simulink model "TVModel"  (R2022a)
settings: Solver=FixedStepDiscrete  StartTime=0.0  StopTime=10.0  FixedStep=0.02  MaxStep=0.01  RelTol=1e-3
undefined symbols (not defined in the file or in its folder): MB, TV, TV_OLD
libraries: simulink x22, simulink_extras x14, slpidlib x8, fuzblock x5, controlLib x4, dspstat3 x4, eeGeneralControl x3, cstblocks x3, eeSlidingModeController x1, sharedTrackingLibrary x1
(part 7 of 8)

== system TVModel/Subsystem/Subsystem1/Torque Distribution/MPC/States Constraints/Tire Bound Dynamics/Slip Angle Calculation/Slip Angle RL ==
  In Bus Element : Inport  PortName=dynamics_data  Element=vy
  In Bus Element1 : Inport  PortName=dynamics_data  Element=vx
  In Bus Element2 : Inport  PortName=dynamics_data  Element=yaw_rate
  In Bus Element3 : Inport  PortName=dynamics_data  Element=yaw_rate
  Atan : Trigonometry  Operator=atan2
  Gain : Gain  Gain=TV.CAR.b
  Gain1 : Gain  Gain=TV.CAR.tr/2
  Subtract : Sum  Inputs=+-
  Subtract1 : Sum  Inputs=+-
  alpha_rl : Outport
  wires:
  In Bus Element2/1 -> Gain/1
  In Bus Element/1 -> Subtract1/1
  In Bus Element3/1 -> Gain1/1
  In Bus Element1/1 -> Subtract/1
  Subtract1/1 -> Atan/1
  Atan/1 -> alpha_rl/1
  Gain1/1 -> Subtract/2
  Gain/1 -> Subtract1/2
  Subtract/1 -> Atan/2

== system TVModel/Subsystem/Subsystem1/Torque Distribution/MPC/States Constraints/Tire Bound Dynamics/Slip Angle Calculation/Slip Angle RR ==
  In Bus Element : Inport  PortName=dynamics_data  Element=vy
  In Bus Element1 : Inport  PortName=dynamics_data  Element=vx
  In Bus Element2 : Inport  PortName=dynamics_data  Element=yaw_rate
  In Bus Element4 : Inport  PortName=dynamics_data  Element=yaw_rate
  Atan : Trigonometry  Operator=atan2
  Gain : Gain  Gain=TV.CAR.b
  Gain1 : Gain  Gain=TV.CAR.tr/2
  Subtract : Sum
  Subtract1 : Sum  Inputs=+-
  alpha_rr : Outport
  wires:
  In Bus Element4/1 -> Gain/1
  In Bus Element/1 -> Subtract1/1
  In Bus Element2/1 -> Gain1/1
  In Bus Element1/1 -> Subtract/1
  Subtract1/1 -> Atan/1
  Atan/1 -> alpha_rr/1
  Gain1/1 -> Subtract/2
  Gain/1 -> Subtract1/2
  Subtract/1 -> Atan/2

== system TVModel/Subsystem/Subsystem1/Torque Distribution/MPC/USEFUL STUFFFF/Power flag/Efficiency limit/Power to engines ==
  omega_motor : Inport
  Torque : Inport  Port=2
  2-D Lookup Table : Lookup_n-D  BreakpointsForDimension1=TV.LV.efficiency_LUT.Omega  BreakpointsForDimension2=TV.LV.efficiency_LUT.Torque  Table=TV.LV.efficiency_LUT.Eta  InternalRulePriority=Speed  RndMeth=Simplest
      settings: InputPortMap=u0,u1
  Abs : Abs  SaturateOnIntegerOverflow=off
  Saturation : Saturate  UpperLimit=1  LowerLimit=0.3
  Efficiency : Outport
  wires:
  Abs/1 -> 2-D Lookup Table/2
  omega_motor/1 -> 2-D Lookup Table/1  "[rad/s]"
  Saturation/1 -> Efficiency/1  "eta_22"
  2-D Lookup Table/1 -> Saturation/1
  Torque/1 -> Abs/1

== system TVModel/Subsystem/Subsystem1/Torque Distribution/MPC/USEFUL STUFFFF/Subsystem1/Steer Activation/First Activation ==
  In1 : Inport
  AND1 : Logic  IconShape=distinctive  AllPortsSameDT=off  OutDataTypeStr=boolean
  Constant9 : Constant  Value=0
  Less Than3 : RelationalOperator  Operator===  OutDataTypeStr=boolean  RndMeth=Simplest  InputSameDT=off
  Less Than4 : RelationalOperator  Operator=<  OutDataTypeStr=boolean  RndMeth=Simplest  InputSameDT=off
  Unit Delay1 : UnitDelay  SampleTime=-1  HasFrameUpgradeWarning=on
  Out1 : Outport
  wires:
  Constant9/1 -> Less Than3/2, Less Than4/1
  Unit Delay1/1 -> Less Than3/1
  In1/1 -> Less Than4/2, Unit Delay1/1
  Less Than4/1 -> AND1/2
  Less Than3/1 -> AND1/1
  AND1/1 -> Out1/1

== system TVModel/Subsystem/Subsystem1/Torque Distribution/MPC/USEFUL STUFFFF/Subsystem1/Steer Activation/If Action Subsystem ==
  Inport : Inport
  Action Port : ActionPort
  Data Type Conversion : DataTypeConversion  OutDataTypeStr=double  RndMeth=Nearest  SaturateOnIntegerOverflow=off
  Epsilon : Outport
  wires:
  Inport/1 -> Data Type Conversion/1
  Data Type Conversion/1 -> Epsilon/1

== system TVModel/Subsystem/Subsystem1/Torque Distribution/MPC/USEFUL STUFFFF/Subsystem1/Steer Activation/If Action Subsystem1 ==
  Inport : Inport
  Action Port : ActionPort
  Constant : Constant  Value=1*pi/180
  Gain : Gain  Gain=1/(2*pi/180)
  Saturation : Saturate  UpperLimit=1  LowerLimit=0
  Saturation1 : Saturate  UpperLimit=inf  LowerLimit=0
  Subtract : Sum  Inputs=+-
  epsilon : Outport
  wires:
  Saturation1/1 -> Gain/1
  Saturation/1 -> epsilon/1
  Gain/1 -> Saturation/1
  Subtract/1 -> Saturation1/1
  Inport/1 -> Subtract/1
  Constant/1 -> Subtract/2

== system TVModel/Subsystem/Subsystem1/Torque Distribution/MPC/ PRE LUDO/Faul Detection/Vectorino/Vectorino/30//70 ==
  In1 : Inport
  Constant2 : Constant  Value=TV.LV.TORQUE.T_peak_motor*[0.3;0.3;1;1]
  Product : Product
  Out1 : Outport
  wires:
  In1/1 -> Product/1
  Product/1 -> Out1/1
  Constant2/1 -> Product/2

== system TVModel/Subsystem/Subsystem1/Torque Distribution/MPC/ PRE LUDO/Faul Detection/Vectorino/Vectorino/Vectorino ==
  In Bus Element4 : Inport  PortName=driver_inputs  Element=steering
  In Bus Element1 : Inport  PortName=driver_inputs  Element=throttle
  In Bus Element : Inport  Port=2  PortName=dynamics_data  Element=omega_wheels
  In Bus Element32 : Inport  Port=3  PortName=brake_signal
  If Action Subsystem2 : Subsystem  TreatAsAtomicUnit=on
  Omega wheels : Subsystem
  Saturation : Saturate  UpperLimit=+inf  LowerLimit=0
  Out Bus Element : Outport  PortName=TV
  wires:
  In Bus Element/1 -> Omega wheels/1(vehBUS)
  In Bus Element1/1 -> If Action Subsystem2/3(Thr)
  In Bus Element32/1 -> If Action Subsystem2/4(Brake)
  Saturation/1 -> If Action Subsystem2/2(Omega wheels)
  In Bus Element4/1 -> If Action Subsystem2/1(delta)
  Omega wheels/1(omega wheels) -> Saturation/1
  If Action Subsystem2/1(T vectorino) -> Out Bus Element/1

== system TVModel/Subsystem/Subsystem1/Torque Distribution/MPC/Faults Detection/Vectorino/Vectorino/Vectorino/If Action Subsystem2 ==
  In Bus Element2 : Inport  PortName=delta
  In Bus Element : Inport  Port=2  PortName=Omega wheels
  In Bus Element1 : Inport  Port=2  PortName=Omega wheels
  In Bus Element5 : Inport  Port=3  PortName=Thr
  In Bus Element3 : Inport  Port=4  PortName=Brake
  In Bus Element4 : Inport  Port=4  PortName=Brake
  If : If  IfExpression=u1 < 0.001
  If Action Subsystem : Subsystem  TreatAsAtomicUnit=on
  If Action Subsystem1 : Subsystem  TreatAsAtomicUnit=on
  Lateral Distribution : Subsystem
  Longitudinal Distribution : Subsystem
  Merge : Merge
  Regen : Subsystem
  T vectorino : Outport
  wires:
  Merge/1 -> T vectorino/1
  If/2 -> If Action Subsystem1/Action
  If/1 -> If Action Subsystem/Action
  In Bus Element2/1 -> Lateral Distribution/2(delta)
  Lateral Distribution/1(TV) -> If Action Subsystem/1(T TV)
  Longitudinal Distribution/1(Front Axle Torque) -> Lateral Distribution/1(Front Axle Torque)
  In Bus Element5/1 -> Longitudinal Distribution/1(Throttle)
  Longitudinal Distribution/2(" Rear Axle Torque") -> Lateral Distribution/3(Rear Axle Torque)
  Regen/1(TV) -> If Action Subsystem1/1(T vectorino)
  If Action Subsystem/1(T_out) -> Merge/1
  If Action Subsystem1/1(T regen) -> Merge/2
  In Bus Element/1 -> Regen/1(Omega wheels)
  In Bus Element1/1 -> Lateral Distribution/4(omega wheels)
  In Bus Element3/1 -> Regen/2(Brake)
  In Bus Element4/1 -> If/1

== system TVModel/Subsystem/Subsystem1/Torque Distribution/MPC/Faults Detection/Vectorino/Vectorino/Vectorino/Omega wheels ==
  In Bus Element : Inport  PortName=vehBUS  Element=Dir.Powertrain.FR.Motor.Velocity
  In Bus Element1 : Inport  PortName=vehBUS  Element=Dir.Powertrain.FL.Motor.Velocity
  In Bus Element2 : Inport  PortName=vehBUS  Element=Dir.Powertrain.RL.Motor.Velocity
  In Bus Element3 : Inport  PortName=vehBUS  Element=Dir.Powertrain.RR.Motor.Velocity
  Gain1 : Gain  Gain=30/pi
  Mux : Mux
  omega wheels : Outport
  wires:
  Gain1/1 -> omega wheels/1
  Mux/1 -> Gain1/1
  In Bus Element1/1 -> Mux/1
  In Bus Element/1 -> Mux/2
  In Bus Element2/1 -> Mux/3
  In Bus Element3/1 -> Mux/4

== system TVModel/Subsystem/Subsystem1/Torque Distribution/MPC/ PRE LUDO/Faul Detection/Vectorino/Vectorino/Vectorino/If Action Subsystem2 ==
  In Bus Element2 : Inport  PortName=delta
  In Bus Element : Inport  Port=2  PortName=Omega wheels
  In Bus Element1 : Inport  Port=2  PortName=Omega wheels
  In Bus Element5 : Inport  Port=3  PortName=Thr
  In Bus Element3 : Inport  Port=4  PortName=Brake
  In Bus Element4 : Inport  Port=4  PortName=Brake
  If : If  IfExpression=u1 < 0.001
  If Action Subsystem : Subsystem  TreatAsAtomicUnit=on
  If Action Subsystem1 : Subsystem  TreatAsAtomicUnit=on
  Lateral Distribution : Subsystem
  Longitudinal Distribution : Subsystem
  Merge : Merge
  Regen : Subsystem
  T vectorino : Outport
  wires:
  In Bus Element4/1 -> If/1
  In Bus Element3/1 -> Regen/2(Brake)
  In Bus Element1/1 -> Lateral Distribution/4(omega wheels)
  In Bus Element/1 -> Regen/1(Omega wheels)
  If Action Subsystem1/1(T regen) -> Merge/2
  If Action Subsystem/1(T_out) -> Merge/1
  Regen/1(TV) -> If Action Subsystem1/1(T vectorino)
  Longitudinal Distribution/2(" Rear Axle Torque") -> Lateral Distribution/3(Rear Axle Torque)
  In Bus Element5/1 -> Longitudinal Distribution/1(Throttle)
  Longitudinal Distribution/1(Front Axle Torque) -> Lateral Distribution/1(Front Axle Torque)
  Lateral Distribution/1(TV) -> If Action Subsystem/1(T TV)
  In Bus Element2/1 -> Lateral Distribution/2(delta)
  If/1 -> If Action Subsystem/Action
  If/2 -> If Action Subsystem1/Action
  Merge/1 -> T vectorino/1

== system TVModel/Subsystem/Subsystem1/Torque Distribution/MPC/ PRE LUDO/Faul Detection/Vectorino/Vectorino/Vectorino/Omega wheels ==
  In Bus Element : Inport  PortName=vehBUS  Element=Dir.Powertrain.FR.Motor.Velocity
  In Bus Element1 : Inport  PortName=vehBUS  Element=Dir.Powertrain.FL.Motor.Velocity
  In Bus Element2 : Inport  PortName=vehBUS  Element=Dir.Powertrain.RL.Motor.Velocity
  In Bus Element3 : Inport  PortName=vehBUS  Element=Dir.Powertrain.RR.Motor.Velocity
  Gain1 : Gain  Gain=30/pi
  Mux : Mux
  omega wheels : Outport
  wires:
  In Bus Element3/1 -> Mux/4
  In Bus Element2/1 -> Mux/3
  In Bus Element/1 -> Mux/2
  In Bus Element1/1 -> Mux/1
  Mux/1 -> Gain1/1
  Gain1/1 -> omega wheels/1

== system TVModel/Subsystem/Subsystem1/Torque Distribution/MPC/Faults Detection/Vectorino/Vectorino/Vectorino/If Action Subsystem2/If Action Subsystem ==
  T TV : Inport
  Action Port : ActionPort
  T_out : Outport
  wires:
  T TV/1 -> T_out/1

== system TVModel/Subsystem/Subsystem1/Torque Distribution/MPC/Faults Detection/Vectorino/Vectorino/Vectorino/If Action Subsystem2/If Action Subsystem1 ==
  T vectorino : Inport
  Action Port : ActionPort
  T regen : Outport
  wires:
  T vectorino/1 -> T regen/1

== system TVModel/Subsystem/Subsystem1/Torque Distribution/MPC/Faults Detection/Vectorino/Vectorino/Vectorino/If Action Subsystem2/Lateral Distribution ==
  Front Axle Torque : Inport
  delta : Inport  Port=2
  Rear Axle Torque : Inport  Port=3
  omega wheels : Inport  Port=4
  "   " : Constant  Value=0.5
  " " : Constant  Value=0.5
  Abs : Abs  SaturateOnIntegerOverflow=off
  Constant4 : Constant  Value=alphaR
  Dynamic Saturation : Subsystem
  FL : Switch  Criteria=u2 > Threshold  SaturateOnIntegerOverflow=off  InputSameDT=off
  FR : Switch  Criteria=u2 > Threshold  SaturateOnIntegerOverflow=off  InputSameDT=off
  Product{1..4} (4 alike) : Product
  RL : Switch  Criteria=u2 > Threshold  SaturateOnIntegerOverflow=off  InputSameDT=off
  RR : Switch  Criteria=u2 > Threshold  SaturateOnIntegerOverflow=off  InputSameDT=off
  Sum : Sum  Inputs=|++
  Sum1 : Sum  Inputs=|+-
  Sum2 : Sum  Inputs=++|
  Sum3 : Sum  Inputs=|+-
  alpha : Constant  Value=alphaF
  TV : Outport
  wires:
  Constant4/1 -> Product4/2
  Sum2/1 -> Product3/1
  Abs/1 -> Product2/2, Product4/1
  Sum/1 -> Product1/2
  " "/1 -> Sum/1
  Product4/1 -> Sum2/1
  Rear Axle Torque/1 -> Sum3/1, Product3/2
  "   "/1 -> Sum2/2
  Product2/1 -> Sum/2
  Product1/1 -> FR/1, FL/3, Sum1/2
  Sum1/1 -> FL/1, FR/3
  alpha/1 -> Product2/1
  delta/1 -> FR/2, FL/2, RL/2, RR/2, Abs/1
  Sum3/1 -> RL/1, RR/3
  Front Axle Torque/1 -> Sum1/1, Product1/1
  Product3/1 -> RR/1, RL/3, Sum3/2
  FL/1 -> Dynamic Saturation/1(T FL)
  FR/1 -> Dynamic Saturation/2(T FR)
  RL/1 -> Dynamic Saturation/4(T RL)
  RR/1 -> Dynamic Saturation/5(T RR)
  omega wheels/1 -> Dynamic Saturation/3(omega wheels)
  Dynamic Saturation/1(TV) -> TV/1

== system TVModel/Subsystem/Subsystem1/Torque Distribution/MPC/Faults Detection/Vectorino/Vectorino/Vectorino/If Action Subsystem2/Longitudinal Distribution ==
  Throttle : Inport
  Add : Sum
  Add1 : Sum  Inputs=+-
  Constant : Constant  Value=T_max*2
  Constant1 : Constant  Value=longR
  Constant2 : Constant  Value=soglia
  Gain4 : Gain  Gain=(maxLongR-longR)/(1-soglia)
  Gain5 : Gain  Gain=longR
  Product1 : Product
  Product2 : Product
  Sum3 : Sum  Inputs=-+|
  Switch : Switch  Criteria=u2 > Threshold  Threshold=T_max*2  SaturateOnIntegerOverflow=off  InputSameDT=off
  Switch1 : Switch  Criteria=u2 > Threshold  Threshold=soglia  SaturateOnIntegerOverflow=off  InputSameDT=off
  "T max " : Constant  Value=T_max*4
  Front Axle Torque : Outport
  " Rear Axle Torque" : Outport  Port=2
  wires:
  Constant1/1 -> Add/2
  Add1/1 -> Gain4/1
  Gain5/1 -> Switch1/3
  Throttle/1 -> Product1/1, Switch1/2, Add1/1
  Gain4/1 -> Add/1
  Add/1 -> Product2/1
  Switch1/1 -> Front Axle Torque/1, Sum3/1
  Switch/1 -> Switch1/1
  Product1/1 -> Gain5/1, Product2/2, Sum3/2
  Sum3/1 -> " Rear Axle Torque"/1
  "T max "/1 -> Product1/2
  Constant2/1 -> Add1/2
  Product2/1 -> Switch/3, Switch/2
  Constant/1 -> Switch/1

== system TVModel/Subsystem/Subsystem1/Torque Distribution/MPC/Faults Detection/Vectorino/Vectorino/Vectorino/If Action Subsystem2/Regen ==
  Omega wheels : Inport
  In Bus Element{,1..3} (4 alike) : Inport  Port=2  PortName=Brake
  1-D Lookup Table{1..4} (4 alike) : Lookup_n-D  NumberOfTableDimensions=1  BreakpointsForDimension1=rpm  Table=torque_regen  InternalRulePriority=Speed  RndMeth=Simplest
  Demux1 : Demux
  Product{9,11,13,15} (4 alike) : Product
  Out Bus Element : Outport  PortName=TV  Element=FL
  Out Bus Element1 : Outport  PortName=TV  Element=FR
  Out Bus Element2 : Outport  PortName=TV  Element=RL
  Out Bus Element3 : Outport  PortName=TV  Element=RR
  wires:
  1-D Lookup Table3/1 -> Product13/2
  1-D Lookup Table1/1 -> Product11/2
  Product15/1 -> Out Bus Element2/1
  Product9/1 -> Out Bus Element/1
  1-D Lookup Table2/1 -> Product15/2
  Product13/1 -> Out Bus Element3/1
  Omega wheels/1 -> Demux1/1
  Demux1/2 -> 1-D Lookup Table1/1
  Demux1/1 -> 1-D Lookup Table4/1
  Product11/1 -> Out Bus Element1/1
  Demux1/3 -> 1-D Lookup Table2/1
  Demux1/4 -> 1-D Lookup Table3/1
  In Bus Element/1 -> Product13/1
  In Bus Element1/1 -> Product15/1
  In Bus Element2/1 -> Product11/1
  In Bus Element3/1 -> Product9/1
  1-D Lookup Table4/1 -> Product9/2

== system TVModel/Subsystem/Subsystem1/Torque Distribution/MPC/ PRE LUDO/Faul Detection/Vectorino/Vectorino/Vectorino/If Action Subsystem2/If Action Subsystem ==
  T TV : Inport
  Action Port : ActionPort
  T_out : Outport
  wires:
  T TV/1 -> T_out/1

== system TVModel/Subsystem/Subsystem1/Torque Distribution/MPC/ PRE LUDO/Faul Detection/Vectorino/Vectorino/Vectorino/If Action Subsystem2/If Action Subsystem1 ==
  T vectorino : Inport
  Action Port : ActionPort
  T regen : Outport
  wires:
  T vectorino/1 -> T regen/1

== system TVModel/Subsystem/Subsystem1/Torque Distribution/MPC/ PRE LUDO/Faul Detection/Vectorino/Vectorino/Vectorino/If Action Subsystem2/Lateral Distribution ==
  Front Axle Torque : Inport
  delta : Inport  Port=2
  Rear Axle Torque : Inport  Port=3
  omega wheels : Inport  Port=4
  "   " : Constant  Value=0.5
  " " : Constant  Value=0.5
  Abs : Abs  SaturateOnIntegerOverflow=off
  Constant4 : Constant  Value=alphaR
  Dynamic Saturation : Subsystem
  FL : Switch  Criteria=u2 > Threshold  SaturateOnIntegerOverflow=off  InputSameDT=off
  FR : Switch  Criteria=u2 > Threshold  SaturateOnIntegerOverflow=off  InputSameDT=off
  Product{1..4} (4 alike) : Product
  RL : Switch  Criteria=u2 > Threshold  SaturateOnIntegerOverflow=off  InputSameDT=off
  RR : Switch  Criteria=u2 > Threshold  SaturateOnIntegerOverflow=off  InputSameDT=off
  Sum : Sum  Inputs=|++
  Sum1 : Sum  Inputs=|+-
  Sum2 : Sum  Inputs=++|
  Sum3 : Sum  Inputs=|+-
  alpha : Constant  Value=alphaF
  TV : Outport
  wires:
  Dynamic Saturation/1(TV) -> TV/1
  omega wheels/1 -> Dynamic Saturation/3(omega wheels)
  RR/1 -> Dynamic Saturation/5(T RR)
  RL/1 -> Dynamic Saturation/4(T RL)
  FR/1 -> Dynamic Saturation/2(T FR)
  FL/1 -> Dynamic Saturation/1(T FL)
  Product3/1 -> Sum3/2, RL/3, RR/1
  Front Axle Torque/1 -> Product1/1, Sum1/1
  Sum3/1 -> RR/3, RL/1
  delta/1 -> Abs/1, RR/2, RL/2, FL/2, FR/2
  alpha/1 -> Product2/1
  Sum1/1 -> FR/3, FL/1
  Product1/1 -> Sum1/2, FL/3, FR/1
  Product2/1 -> Sum/2
  "   "/1 -> Sum2/2
  Rear Axle Torque/1 -> Product3/2, Sum3/1
  Product4/1 -> Sum2/1
  " "/1 -> Sum/1
  Sum/1 -> Product1/2
  Abs/1 -> Product4/1, Product2/2
  Sum2/1 -> Product3/1
  Constant4/1 -> Product4/2

== system TVModel/Subsystem/Subsystem1/Torque Distribution/MPC/ PRE LUDO/Faul Detection/Vectorino/Vectorino/Vectorino/If Action Subsystem2/Longitudinal Distribution ==
  Throttle : Inport
  Add : Sum
  Add1 : Sum  Inputs=+-
  Constant : Constant  Value=T_max*2
  Constant1 : Constant  Value=longR
  Constant2 : Constant  Value=soglia
  Gain4 : Gain  Gain=(maxLongR-longR)/(1-soglia)
  Gain5 : Gain  Gain=longR
  Product1 : Product
  Product2 : Product
  Sum3 : Sum  Inputs=-+|
  Switch : Switch  Criteria=u2 > Threshold  Threshold=T_max*2  SaturateOnIntegerOverflow=off  InputSameDT=off
  Switch1 : Switch  Criteria=u2 > Threshold  Threshold=soglia  SaturateOnIntegerOverflow=off  InputSameDT=off
  "T max " : Constant  Value=T_max*4
  Front Axle Torque : Outport
  " Rear Axle Torque" : Outport  Port=2
  wires:
  Constant/1 -> Switch/1
  Product2/1 -> Switch/2, Switch/3
  Constant2/1 -> Add1/2
  "T max "/1 -> Product1/2
  Sum3/1 -> " Rear Axle Torque"/1
  Product1/1 -> Sum3/2, Product2/2, Gain5/1
  Switch/1 -> Switch1/1
  Switch1/1 -> Sum3/1, Front Axle Torque/1
  Add/1 -> Product2/1
  Gain4/1 -> Add/1
  Throttle/1 -> Add1/1, Switch1/2, Product1/1
  Gain5/1 -> Switch1/3
  Add1/1 -> Gain4/1
  Constant1/1 -> Add/2

== system TVModel/Subsystem/Subsystem1/Torque Distribution/MPC/ PRE LUDO/Faul Detection/Vectorino/Vectorino/Vectorino/If Action Subsystem2/Regen ==
  Omega wheels : Inport
  In Bus Element{,1..3} (4 alike) : Inport  Port=2  PortName=Brake
  1-D Lookup Table{1..4} (4 alike) : Lookup_n-D  NumberOfTableDimensions=1  BreakpointsForDimension1=rpm  Table=torque_regen  InternalRulePriority=Speed  RndMeth=Simplest
  Demux1 : Demux
  Product{9,11,13,15} (4 alike) : Product
  Out Bus Element : Outport  PortName=TV  Element=FL
  Out Bus Element1 : Outport  PortName=TV  Element=FR
  Out Bus Element2 : Outport  PortName=TV  Element=RL
  Out Bus Element3 : Outport  PortName=TV  Element=RR
  wires:
  1-D Lookup Table4/1 -> Product9/2
  In Bus Element3/1 -> Product9/1
  In Bus Element2/1 -> Product11/1
  In Bus Element1/1 -> Product15/1
  In Bus Element/1 -> Product13/1
  Demux1/4 -> 1-D Lookup Table3/1
  Demux1/3 -> 1-D Lookup Table2/1
  Product11/1 -> Out Bus Element1/1
  Demux1/1 -> 1-D Lookup Table4/1
  Demux1/2 -> 1-D Lookup Table1/1
  Omega wheels/1 -> Demux1/1
  Product13/1 -> Out Bus Element3/1
  1-D Lookup Table2/1 -> Product15/2
  Product9/1 -> Out Bus Element/1
  Product15/1 -> Out Bus Element2/1
  1-D Lookup Table1/1 -> Product11/2
  1-D Lookup Table3/1 -> Product13/2

== system TVModel/Subsystem/Subsystem1/Torque Distribution/MPC/Faults Detection/Vectorino/Vectorino/Vectorino/If Action Subsystem2/Lateral Distribution/Dynamic Saturation ==
  T FL : Inport
  T FR : Inport  Port=2
  omega wheels : Inport  Port=3
  T RL : Inport  Port=4
  T RR : Inport  Port=5
  1-D Lookup Table{,1..3} (4 alike) : Lookup_n-D  NumberOfTableDimensions=1  BreakpointsForDimension1=rpm  Table=torque  InternalRulePriority=Speed  RndMeth=Simplest
  Constant{,1..3} (4 alike) : Constant  Value=0
  Demux : Demux
  Saturation Dynamic{,1..3} (4 alike) : simulink/Discontinuities/Saturation Dynamic  OutMin=[]  OutMax=[]  OutDataTypeStr=Inherit: Same as second input  OutDataType=fixdt(1, 16)  OutScaling=2^-10  DoSatur=off
  Out Bus Element : Outport  PortName=TV  Element=FL
  Out Bus Element1 : Outport  PortName=TV  Element=FR
  Out Bus Element2 : Outport  PortName=TV  Element=RL
  Out Bus Element3 : Outport  PortName=TV  Element=RR
  wires:
  Demux/1 -> 1-D Lookup Table/1
  Saturation Dynamic/1 -> Out Bus Element/1
  Constant3/1 -> Saturation Dynamic3/3
  1-D Lookup Table2/1 -> Saturation Dynamic2/1
  Saturation Dynamic3/1 -> Out Bus Element3/1
  Saturation Dynamic1/1 -> Out Bus Element1/1
  1-D Lookup Table/1 -> Saturation Dynamic/1
  Constant2/1 -> Saturation Dynamic2/3
  1-D Lookup Table3/1 -> Saturation Dynamic3/1
  Constant1/1 -> Saturation Dynamic1/3
  1-D Lookup Table1/1 -> Saturation Dynamic1/1
  Saturation Dynamic2/1 -> Out Bus Element2/1
  Constant/1 -> Saturation Dynamic/3
  Demux/2 -> 1-D Lookup Table1/1
  T RL/1 -> Saturation Dynamic2/2
  T RR/1 -> Saturation Dynamic3/2
  T FL/1 -> Saturation Dynamic/2
  T FR/1 -> Saturation Dynamic1/2
  Demux/4 -> 1-D Lookup Table3/1
  Demux/3 -> 1-D Lookup Table2/1
  omega wheels/1 -> Demux/1

== system TVModel/Subsystem/Subsystem1/Torque Distribution/MPC/ PRE LUDO/Faul Detection/Vectorino/Vectorino/Vectorino/If Action Subsystem2/Lateral Distribution/Dynamic Saturation ==
  T FL : Inport
  T FR : Inport  Port=2
  omega wheels : Inport  Port=3
  T RL : Inport  Port=4
  T RR : Inport  Port=5
  1-D Lookup Table{,1..3} (4 alike) : Lookup_n-D  NumberOfTableDimensions=1  BreakpointsForDimension1=rpm  Table=torque  InternalRulePriority=Speed  RndMeth=Simplest
  Constant{,1..3} (4 alike) : Constant  Value=0
  Demux : Demux
  Saturation Dynamic{,1..3} (4 alike) : simulink/Discontinuities/Saturation Dynamic  OutMin=[]  OutMax=[]  OutDataTypeStr=Inherit: Same as second input  OutDataType=fixdt(1, 16)  OutScaling=2^-10  DoSatur=off
  Out Bus Element : Outport  PortName=TV  Element=FL
  Out Bus Element1 : Outport  PortName=TV  Element=FR
  Out Bus Element2 : Outport  PortName=TV  Element=RL
  Out Bus Element3 : Outport  PortName=TV  Element=RR
  wires:
  omega wheels/1 -> Demux/1
  Demux/3 -> 1-D Lookup Table2/1
  Demux/4 -> 1-D Lookup Table3/1
  T FR/1 -> Saturation Dynamic1/2
  T FL/1 -> Saturation Dynamic/2
  T RR/1 -> Saturation Dynamic3/2
  T RL/1 -> Saturation Dynamic2/2
  Demux/2 -> 1-D Lookup Table1/1
  Constant/1 -> Saturation Dynamic/3
  Saturation Dynamic2/1 -> Out Bus Element2/1
  1-D Lookup Table1/1 -> Saturation Dynamic1/1
  Constant1/1 -> Saturation Dynamic1/3
  1-D Lookup Table3/1 -> Saturation Dynamic3/1
  Constant2/1 -> Saturation Dynamic2/3
  1-D Lookup Table/1 -> Saturation Dynamic/1
  Saturation Dynamic1/1 -> Out Bus Element1/1
  Saturation Dynamic3/1 -> Out Bus Element3/1
  1-D Lookup Table2/1 -> Saturation Dynamic2/1
  Constant3/1 -> Saturation Dynamic3/3
  Saturation Dynamic/1 -> Out Bus Element/1
  Demux/1 -> 1-D Lookup Table/1

== matlab function TVModel/Subsystem/Subsystem1/Slip Control/Traction Control/MATLAB Function ==
  data: u input; y output
function y = fcn(u)


% @(Fz,LMUX,kappa)
muX = ((Fz.^2.*LMUX)./1.0e+4-Fz.*LMUX.*sin(atan((Fz.*5.946e-5-6.5736e-1).*(sign(Fz.*(-1.5696e-6)+kappa+6.665e-4).*5.242e-1+1.0).*(atan((Fz.*exp(Fz.*(-1.3455e-5)+1.3455e-2).*(Fz.*(3.0./2.0e+2)+6.77e+2./1.0e+1).*(Fz.*(-1.5696e-6)+kappa+6.665e-4).*(3.33e+2./4.0e+2))./(Fz.*LMUX.*2.5847808+1.0./1.0e+2))-(Fz.*exp(Fz.*(-1.3455e-5)+1.3455e-2).*(Fz.*(3.0./2.0e+2)+6.77e+2./1.0e+1).*(Fz.*(-1.5696e-6)+kappa+6.665e-4).*(3.33e+2./4.0e+2))./(Fz.*LMUX.*2.5847808+1.0./1.0e+2))-(Fz.*exp(Fz.*(-1.3455e-5)+1.3455e-2).*(Fz.*(3.0./2.0e+2)+6.77e+2./1.0e+1).*(Fz.*(-1.5696e-6)+kappa+6.665e-4).*(3.33e+2./4.0e+2))./(Fz.*LMUX.*2.5847808+1.0./1.0e+2)).*(1.68e+2./1.25e+2)).*1.9232)./Fz

y = u;

== matlab function TVModel/Subsystem/Subsystem1/Torque Distribution/MPC/ PRE LUDO/Cross Check1 ==
  data: ubu input; param input; ubu output; lbu input; lbu output
function [ubu,lbu] = fcn(ubu,param,lbu)
flag = param(1);
ubu_target = param(2:5);
lbu_target = param(6:9);
lbu_max = param(10);
switch flag
    case 0 %% Check cross between bounds
        for i = 1 : 4
            if lbu(i) > ubu(i)
               lbu(i) = ubu(i) - lbu_max;
            end
        end
    case 1 %% Check for low YRD Accelerating
        for i = 1 :4
            ubu(i) = ubu_target(i);
            lbu(i) = 0;
        end
    case 2 %% Check for low YRD Braking
        for i = 1:4
            lbu(i) = lbu_target(i);
            ubu(i) = 0;
        end
    case 3 %% Overlapping
        for i = 1:4
            lbu(i) = 0;
            ubu(i) = 0;
        end
end

== matlab function TVModel/Subsystem/Subsystem1/Torque Distribution/MPC/Mz Generation/MATLAB Function1 ==
  data: Mz input; lbMz output; ubMz output
function [lbMz,ubMz] = fcn(Mz)

lb = 0.25;
ub = 1.1;

if sign(Mz) > 0
   lbMz = Mz*lb;
   ubMz = Mz*ub;
else
   lbMz = Mz*ub;
   ubMz = Mz*lb;
end

== matlab function TVModel/Subsystem/Subsystem1/Torque Distribution/MPC/USEFUL STUFFFF/Extended Kalman Filter/state_update_kalman_simulink/f(x,u) ==
  data: x input; u input; xout output
function xout = state_update_kalman_simulink(x,u)

%% ~~~~~~~~~~~~~~~~~~~~~~~~~~~~~ Intro ~~~~~~~~~~~~~~~~~~~~~~~~~~~~~~~~~~~~
dt = 1/50;
%% ~~~~~~~~~~~~~~~~~~~~~~~~ Car parameters ~~~~~~~~~~~~~~~~~~~~~~~~~~~~~~~~
xout = zeros(3,1);
% ~~~~~~~~~~~~~~~~~~~~~~~~ General Parameters ~~~~~~~~~~~~~~~~~~~~~~~~~~~~~
g   = 9.81;            % [m/s^2]                          
wd  = 0.5;             % [~]         
wb  = 1.53;            % [~]          
tf  = 1.27;            % [m]          
tr  = 1.27;            % [m]          
m   = 195+75;          % [Kg]            
Iz  = 120;             % [Kg*m^2]         
a   = wb*wd;           % [m]            
b   = wb - a;          % [m]            
hcog = 0.29;           % [m]           
Fzf  = m*g/2*(wd);     % [N]                 
Fzr  = m*g/2*(1-wd);   % [N]                   
tau = 13.5;            % [~]          
rs  = 0.235;           % [m]           

% ~~~~~~~~~~~~~~~~~~~~~~~~~~~ Aero parameters ~~~~~~~~~~~~~~~~~~~~~~~~~~~~~
wbaero = 0.5542;       % [~]           
hcop = 0.576;          % [m]      
rho = 1.225;           % [Kg/m^3]     
CdA = 1.708;           % [m]     
ClA = 5.14;            % [m]    

% ~~~~~~~~~~~~~~~~~~~~~~~~~~ Other parameters ~~~~~~~~~~~~~~~~~~~~~~~~~~~~~

% ~~~~~~~~~~~~~~~~~~~~~~~~~~~ Set up states  ~~~~~~~~~~~~~~~~~~~~~~~~~~~~~~
vx = x(1);
vy = x(2);
r  = x(3);

% ~~~~~~~~~~~~~~~~~~~~~~~~~~~ Set up parameters ~~~~~~~~~~~~~~~~~~~~~~~~~~~
% delta    = u(1);
% kappa_FL = u(2);
% kappa_FR = u(3);
% kappa_RL = u(4);
% kappa_RR = u(5);
% Tbrk_FL  = u(6);
% Tbrk_FR  = u(7);
% Tbrk_RL  = u(8);
% Tbrk_RR  = u(9);
% ay       = u(10);
% ax       = u(11);
% T_FL     = u(12);
% T_FR     = u(13);
% T_RL     = u(14);
% T_RR     = u(15);

delta    = u(1);
kappa_FL = u(2);
kappa_FR = u(3);
kappa_RL = u(4);
kappa_RR = u(5);
T_FL     = u(6);
T_FR     = u(7);
T_RL     = u(8);
T_RR     = u(9);

ax = 0; ay = 0;
Tbrk_FL  = 0;
Tbrk_FR  = 0;
Tbrk_RL  = 0;
Tbrk_RR  = 0;
%% ~~~~~~~~~~~~~~~~~~~~~~~~~~ System Dynamics ~~~~~~~~~~~~~~~~~~~~~~~~~~~~~~

% ~~~~~~~~~~~~~~~~~~~~~~~~~~~ Aerodynamics ~~~~~~~~~~~~~~~~~~~~~~~~~~~~~~~~
Faerox = 0.5*rho*CdA*vx^2;
Faeroz = 0.5*rho*ClA*vx^2;

% ~~~~~~~~~~~~~~~~~~~~~~~~~~~ Slip Angles ~~~~~~~~~~~~~~~~~~~~~~~~~~~~~~~~~
alpha_FL =  (((vy + r*a)./(vx - r*tf/2)) - delta);
alpha_FR =  (((vy + r*a)./(vx + r*tf/2)) - delta);
alpha_RL =  (((vy - r*b)./(vx - r*tr/2)));     
alpha_RR =  (((vy - r*b)./(vx + r*tr/2)));     

% ~~~~~~~~~~~~~~~~~~~~~~~~~~~ Vertical loads ~~~~~~~~~~~~~~~~~~~~~~~~~~~~~~
Fz_FL = Fzf - 0.5*(m/tf*hcog).*ay + 0.5*Faeroz*wbaero - 0.5*Faerox/wb*hcop - 0.5*(m/wb*hcog).*ax;
Fz_FR = Fzf + 0.5*(m/tf*hcog).*ay + 0.5*Faeroz*wbaero - 0.5*Faerox/wb*hcop - 0.5*(m/wb*hcog).*ax;
Fz_RL = Fzr - 0.5*(m/tr*hcog).*ay + 0.5*Faeroz*(1-wbaero) + 0.5*Faerox/wb*hcop + 0.5*(m/wb*hcog).*ax;
Fz_RR = Fzr + 0.5*(m/tr*hcog).*ay + 0.5*Faeroz*(1-wbaero) + 0.5*Faerox/wb*hcop + 0.5*(m/wb*hcog).*ax;

% ~~~~~~~~~~~~~~~~~~~~~~~~~~ Lateral forces ~~~~~~~~~~~~~~~~~~~~~~~~~~~~~~~
muY = 1.5;
Fy_FL = (cos(0.95064*atan((41.4696*(kappa_FL - 0.00000078224999999999995925481499625675*Fz_FL + 0.00056678999999999995877686398415563))/((13.456699999999999661781657778192*alpha_FL - 0.51027806399999998717476046294905)^2 + 1.0)^(1/2) + (0.0012906*Fz_FL - 2.3215)*(atan((41.4696*(kappa_FL - 0.00000078224999999999995925481499625675*Fz_FL + 0.00056678999999999995877686398415563))/((13.456699999999999661781657778192*alpha_FL - 0.51027806399999998717476046294905)^2 + 1.0)^(1/2)) - (41.4696*(kappa_FL - 0.00000078224999999999995925481499625675*Fz_FL + 0.00056678999999999995877686398415563))/((13.456699999999999661781657778192*alpha_FL - 0.51027806399999998717476046294905)^2 + 1.0)^(1/2))))*(0.93*Fz_FL*(0.000071017999999999997795541162304289*Fz_FL - 0.14887799999999999779554116230429) - 0.93*Fz_FL*(0.00074656*Fz_FL + 0.37814) + Fz_FL*muY*sin(1.1962*atan((28888.097815192522084544179961085*sin(2.0*atan(0.00077863498204218704389788477193347*Fz_FL))*(0.000001140900000000000030428437547414*Fz_FL - 1.0*alpha_FL + (0.93*Fz_FL*(0.00074656*Fz_FL + 0.37814) + 1.1538900000000000822808488010196*Fz_FL*(0.00023917*Fz_FL - 1.57477))/(28888.097815192522084544179961085*sin(2.0*atan(0.00077863498204218704389788477193347*Fz_FL)) - 0.01) + 0.0023905000000000000467265115489113))/(1.1962*Fz_FL*muY + 0.01) - 1.0*(atan((28888.097815192522084544179961085*sin(2.0*atan(0.00077863498204218704389788477193347*Fz_FL))*(0.000001140900000000000030428437547414*Fz_FL - 1.0*alpha_FL + (0.93*Fz_FL*(0.00074656*Fz_FL + 0.37814) + 1.1538900000000000822808488010196*Fz_FL*(0.00023917*Fz_FL - 1.57477))/(28888.097815192522084544179961085*sin(2.0*atan(0.00077863498204218704389788477193347*Fz_FL)) - 0.01) + 0.0023905000000000000467265115489113))/(1.1962*Fz_FL*muY + 0.01)) - (28888.097815192522084544179961085*sin(2.0*atan(0.00077863498204218704389788477193347*Fz_FL))*(0.000001140900000000000030428437547414*Fz_FL - 1.0*alpha_FL + (0.93*Fz_FL*(0.00074656*Fz_FL + 0.37814) + 1.1538900000000000822808488010196*Fz_FL*(0.00023917*Fz_FL - 1.57477))/(28888.097815192522084544179961085*sin(2.0*atan(0.00077863498204218704389788477193347*Fz_FL)) - 0.01) + 0.0023905000000000000467265115489113))/(1.1962*Fz_FL*muY + 0.01))*(0.000039933999999999997276844965199416*Fz_FL - 0.52068399999999999727684496519942)*(0.47036*sign(0.000001140900000000000030428437547414*Fz_FL - 1.0*alpha_FL + (0.93*Fz_FL*(0.00074656*Fz_FL + 0.37814) + 1.1538900000000000822808488010196*Fz_FL*(0.00023917*Fz_FL - 1.57477))/(28888.097815192522084544179961085*sin(2.0*atan(0.00077863498204218704389788477193347*Fz_FL)) - 0.01) + 0.0023905000000000000467265115489113) - 7.9286)))))/cos(0.95064*atan((41.4696*(0.00000078224999999999995925481499625675*Fz_FL - 0.00056678999999999995877686398415563))/((13.456699999999999661781657778192*alpha_FL - 0.51027806399999998717476046294905)^2 + 1.0)^(1/2) + (0.0012906*Fz_FL - 2.3215)*(atan((41.4696*(0.00000078224999999999995925481499625675*Fz_FL - 0.00056678999999999995877686398415563))/((13.456699999999999661781657778192*alpha_FL - 0.51027806399999998717476046294905)^2 + 1.0)^(1/2)) - (41.4696*(0.00000078224999999999995925481499625675*Fz_FL - 0.00056678999999999995877686398415563))/((13.456699999999999661781657778192*alpha_FL - 0.51027806399999998717476046294905)^2 + 1.0)^(1/2)))) - (1.0*Fz_FL*muY*sin(1.9085*atan(16.5046*kappa_FL))*(0.0000027179999999999999299449271461526*Fz_FL - 1.1553830000000000000737188088351))/(225.17103248999997449603881705116*alpha_FL^2 + 1.0)^(1/2) + 400;
Fy_FR = (cos(0.95064*atan((41.4696*(kappa_FR - 0.00000078224999999999995925481499625675*Fz_FR + 0.00056678999999999995877686398415563))/((13.456699999999999661781657778192*alpha_FR - 0.51027806399999998717476046294905)^2 + 1.0)^(1/2) + (0.0012906*Fz_FR - 2.3215)*(atan((41.4696*(kappa_FR - 0.00000078224999999999995925481499625675*Fz_FR + 0.00056678999999999995877686398415563))/((13.456699999999999661781657778192*alpha_FR - 0.51027806399999998717476046294905)^2 + 1.0)^(1/2)) - (41.4696*(kappa_FR - 0.00000078224999999999995925481499625675*Fz_FR + 0.00056678999999999995877686398415563))/((13.456699999999999661781657778192*alpha_FR - 0.51027806399999998717476046294905)^2 + 1.0)^(1/2))))*(0.93*Fz_FR*(0.000071017999999999997795541162304289*Fz_FR - 0.14887799999999999779554116230429) - 0.93*Fz_FR*(0.00074656*Fz_FR + 0.37814) + Fz_FR*muY*sin(1.1962*atan((28888.097815192522084544179961085*sin(2.0*atan(0.00077863498204218704389788477193347*Fz_FR))*(0.000001140900000000000030428437547414*Fz_FR - 1.0*alpha_FR + (0.93*Fz_FR*(0.00074656*Fz_FR + 0.37814) + 1.1538900000000000822808488010196*Fz_FR*(0.00023917*Fz_FR - 1.57477))/(28888.097815192522084544179961085*sin(2.0*atan(0.00077863498204218704389788477193347*Fz_FR)) - 0.01) + 0.0023905000000000000467265115489113))/(1.1962*Fz_FR*muY + 0.01) - 1.0*(atan((28888.097815192522084544179961085*sin(2.0*atan(0.00077863498204218704389788477193347*Fz_FR))*(0.000001140900000000000030428437547414*Fz_FR - 1.0*alpha_FR + (0.93*Fz_FR*(0.00074656*Fz_FR + 0.37814) + 1.1538900000000000822808488010196*Fz_FR*(0.00023917*Fz_FR - 1.57477))/(28888.097815192522084544179961085*sin(2.0*atan(0.00077863498204218704389788477193347*Fz_FR)) - 0.01) + 0.0023905000000000000467265115489113))/(1.1962*Fz_FR*muY + 0.01)) - (28888.097815192522084544179961085*sin(2.0*atan(0.00077863498204218704389788477193347*Fz_FR))*(0.000001140900000000000030428437547414*Fz_FR - 1.0*alpha_FR + (0.93*Fz_FR*(0.00074656*Fz_FR + 0.37814) + 1.1538900000000000822808488010196*Fz_FR*(0.00023917*Fz_FR - 1.57477))/(28888.097815192522084544179961085*sin(2.0*atan(0.00077863498204218704389788477193347*Fz_FR)) - 0.01) + 0.0023905000000000000467265115489113))/(1.1962*Fz_FR*muY + 0.01))*(0.000039933999999999997276844965199416*Fz_FR - 0.52068399999999999727684496519942)*(0.47036*sign(0.000001140900000000000030428437547414*Fz_FR - 1.0*alpha_FR + (0.93*Fz_FR*(0.00074656*Fz_FR + 0.37814) + 1.1538900000000000822808488010196*Fz_FR*(0.00023917*Fz_FR - 1.57477))/(28888.097815192522084544179961085*sin(2.0*atan(0.00077863498204218704389788477193347*Fz_FR)) - 0.01) + 0.0023905000000000000467265115489113) - 7.9286)))))/cos(0.95064*atan((41.4696*(0.00000078224999999999995925481499625675*Fz_FR - 0.00056678999999999995877686398415563))/((13.456699999999999661781657778192*alpha_FR - 0.51027806399999998717476046294905)^2 + 1.0)^(1/2) + (0.0012906*Fz_FR - 2.3215)*(atan((41.4696*(0.00000078224999999999995925481499625675*Fz_FR - 0.00056678999999999995877686398415563))/((13.456699999999999661781657778192*alpha_FR - 0.51027806399999998717476046294905)^2 + 1.0)^(1/2)) - (41.4696*(0.00000078224999999999995925481499625675*Fz_FR - 0.00056678999999999995877686398415563))/((13.456699999999999661781657778192*alpha_FR - 0.51027806399999998717476046294905)^2 + 1.0)^(1/2)))) - (1.0*Fz_FR*muY*sin(1.9085*atan(16.5046*kappa_FR))*(0.0000027179999999999999299449271461526*Fz_FR - 1.1553830000000000000737188088351))/(225.17103248999997449603881705116*alpha_FR^2 + 1.0)^(1/2) + 400;
Fy_RL = (cos(0.95064*atan((41.4696*(kappa_RL - 0.00000078224999999999995925481499625675*Fz_RL + 0.00056678999999999995877686398415563))/((13.456699999999999661781657778192*alpha_RL - 0.51027806399999998717476046294905)^2 + 1.0)^(1/2) + (0.0012906*Fz_RL - 2.3215)*(atan((41.4696*(kappa_RL - 0.00000078224999999999995925481499625675*Fz_RL + 0.00056678999999999995877686398415563))/((13.456699999999999661781657778192*alpha_RL - 0.51027806399999998717476046294905)^2 + 1.0)^(1/2)) - (41.4696*(kappa_RL - 0.00000078224999999999995925481499625675*Fz_RL + 0.00056678999999999995877686398415563))/((13.456699999999999661781657778192*alpha_RL - 0.51027806399999998717476046294905)^2 + 1.0)^(1/2))))*(0.93*Fz_RL*(0.000071017999999999997795541162304289*Fz_RL - 0.14887799999999999779554116230429) - 0.93*Fz_RL*(0.00074656*Fz_RL + 0.37814) + Fz_RL*muY*sin(1.1962*atan((28888.097815192522084544179961085*sin(2.0*atan(0.00077863498204218704389788477193347*Fz_RL))*(0.000001140900000000000030428437547414*Fz_RL - 1.0*alpha_RL + (0.93*Fz_RL*(0.00074656*Fz_RL + 0.37814) + 1.1538900000000000822808488010196*Fz_RL*(0.00023917*Fz_RL - 1.57477))/(28888.097815192522084544179961085*sin(2.0*atan(0.00077863498204218704389788477193347*Fz_RL)) - 0.01) + 0.0023905000000000000467265115489113))/(1.1962*Fz_RL*muY + 0.01) - 1.0*(atan((28888.097815192522084544179961085*sin(2.0*atan(0.00077863498204218704389788477193347*Fz_RL))*(0.000001140900000000000030428437547414*Fz_RL - 1.0*alpha_RL + (0.93*Fz_RL*(0.00074656*Fz_RL + 0.37814) + 1.1538900000000000822808488010196*Fz_RL*(0.00023917*Fz_RL - 1.57477))/(28888.097815192522084544179961085*sin(2.0*atan(0.00077863498204218704389788477193347*Fz_RL)) - 0.01) + 0.0023905000000000000467265115489113))/(1.1962*Fz_RL*muY + 0.01)) - (28888.097815192522084544179961085*sin(2.0*atan(0.00077863498204218704389788477193347*Fz_RL))*(0.000001140900000000000030428437547414*Fz_RL - 1.0*alpha_RL + (0.93*Fz_RL*(0.00074656*Fz_RL + 0.37814) + 1.1538900000000000822808488010196*Fz_RL*(0.00023917*Fz_RL - 1.57477))/(28888.097815192522084544179961085*sin(2.0*atan(0.00077863498204218704389788477193347*Fz_RL)) - 0.01) + 0.0023905000000000000467265115489113))/(1.1962*Fz_RL*muY + 0.01))*(0.000039933999999999997276844965199416*Fz_RL - 0.52068399999999999727684496519942)*(0.47036*sign(0.000001140900000000000030428437547414*Fz_RL - 1.0*alpha_RL + (0.93*Fz_RL*(0.00074656*Fz_RL + 0.37814) + 1.1538900000000000822808488010196*Fz_RL*(0.00023917*Fz_RL - 1.57477))/(28888.097815192522084544179961085*sin(2.0*atan(0.00077863498204218704389788477193347*Fz_RL)) - 0.01) + 0.0023905000000000000467265115489113) - 7.9286)))))/cos(0.95064*atan((41.4696*(0.00000078224999999999995925481499625675*Fz_RL - 0.00056678999999999995877686398415563))/((13.456699999999999661781657778192*alpha_RL - 0.51027806399999998717476046294905)^2 + 1.0)^(1/2) + (0.0012906*Fz_RL - 2.3215)*(atan((41.4696*(0.00000078224999999999995925481499625675*Fz_RL - 0.00056678999999999995877686398415563))/((13.456699999999999661781657778192*alpha_RL - 0.51027806399999998717476046294905)^2 + 1.0)^(1/2)) - (41.4696*(0.00000078224999999999995925481499625675*Fz_RL - 0.00056678999999999995877686398415563))/((13.456699999999999661781657778192*alpha_RL - 0.51027806399999998717476046294905)^2 + 1.0)^(1/2)))) - (1.0*Fz_RL*muY*sin(1.9085*atan(16.5046*kappa_RL))*(0.0000027179999999999999299449271461526*Fz_RL - 1.1553830000000000000737188088351))/(225.17103248999997449603881705116*alpha_RL^2 + 1.0)^(1/2) + 400;
Fy_RR = (cos(0.95064*atan((41.4696*(kappa_RR - 0.00000078224999999999995925481499625675*Fz_RR + 0.00056678999999999995877686398415563))/((13.456699999999999661781657778192*alpha_RR - 0.51027806399999998717476046294905)^2 + 1.0)^(1/2) + (0.0012906*Fz_RR - 2.3215)*(atan((41.4696*(kappa_RR - 0.00000078224999999999995925481499625675*Fz_RR + 0.00056678999999999995877686398415563))/((13.456699999999999661781657778192*alpha_RR - 0.51027806399999998717476046294905)^2 + 1.0)^(1/2)) - (41.4696*(kappa_RR - 0.00000078224999999999995925481499625675*Fz_RR + 0.00056678999999999995877686398415563))/((13.456699999999999661781657778192*alpha_RR - 0.51027806399999998717476046294905)^2 + 1.0)^(1/2))))*(0.93*Fz_RR*(0.000071017999999999997795541162304289*Fz_RR - 0.14887799999999999779554116230429) - 0.93*Fz_RR*(0.00074656*Fz_RR + 0.37814) + Fz_RR*muY*sin(1.1962*atan((28888.097815192522084544179961085*sin(2.0*atan(0.00077863498204218704389788477193347*Fz_RR))*(0.000001140900000000000030428437547414*Fz_RR - 1.0*alpha_RR + (0.93*Fz_RR*(0.00074656*Fz_RR + 0.37814) + 1.1538900000000000822808488010196*Fz_RR*(0.00023917*Fz_RR - 1.57477))/(28888.097815192522084544179961085*sin(2.0*atan(0.00077863498204218704389788477193347*Fz_RR)) - 0.01) + 0.0023905000000000000467265115489113))/(1.1962*Fz_RR*muY + 0.01) - 1.0*(atan((28888.097815192522084544179961085*sin(2.0*atan(0.00077863498204218704389788477193347*Fz_RR))*(0.000001140900000000000030428437547414*Fz_RR - 1.0*alpha_RR + (0.93*Fz_RR*(0.00074656*Fz_RR + 0.37814) + 1.1538900000000000822808488010196*Fz_RR*(0.00023917*Fz_RR - 1.57477))/(28888.097815192522084544179961085*sin(2.0*atan(0.00077863498204218704389788477193347*Fz_RR)) - 0.01) + 0.0023905000000000000467265115489113))/(1.1962*Fz_RR*muY + 0.01)) - (28888.097815192522084544179961085*sin(2.0*atan(0.00077863498204218704389788477193347*Fz_RR))*(0.000001140900000000000030428437547414*Fz_RR - 1.0*alpha_RR + (0.93*Fz_RR*(0.00074656*Fz_RR + 0.37814) + 1.1538900000000000822808488010196*Fz_RR*(0.00023917*Fz_RR - 1.57477))/(28888.097815192522084544179961085*sin(2.0*atan(0.00077863498204218704389788477193347*Fz_RR)) - 0.01) + 0.0023905000000000000467265115489113))/(1.1962*Fz_RR*muY + 0.01))*(0.000039933999999999997276844965199416*Fz_RR - 0.52068399999999999727684496519942)*(0.47036*sign(0.000001140900000000000030428437547414*Fz_RR - 1.0*alpha_RR + (0.93*Fz_RR*(0.00074656*Fz_RR + 0.37814) + 1.1538900000000000822808488010196*Fz_RR*(0.00023917*Fz_RR - 1.57477))/(28888.097815192522084544179961085*sin(2.0*atan(0.00077863498204218704389788477193347*Fz_RR)) - 0.01) + 0.0023905000000000000467265115489113) - 7.9286)))))/cos(0.95064*atan((41.4696*(0.00000078224999999999995925481499625675*Fz_RR - 0.00056678999999999995877686398415563))/((13.456699999999999661781657778192*alpha_RR - 0.51027806399999998717476046294905)^2 + 1.0)^(1/2) + (0.0012906*Fz_RR - 2.3215)*(atan((41.4696*(0.00000078224999999999995925481499625675*Fz_RR - 0.00056678999999999995877686398415563))/((13.456699999999999661781657778192*alpha_RR - 0.51027806399999998717476046294905)^2 + 1.0)^(1/2)) - (41.4696*(0.00000078224999999999995925481499625675*Fz_RR - 0.00056678999999999995877686398415563))/((13.456699999999999661781657778192*alpha_RR - 0.51027806399999998717476046294905)^2 + 1.0)^(1/2)))) - (1.0*Fz_RR*muY*sin(1.9085*atan(16.5046*kappa_RR))*(0.0000027179999999999999299449271461526*Fz_RR - 1.1553830000000000000737188088351))/(225.17103248999997449603881705116*alpha_RR^2 + 1.0)^(1/2) + 400;

% ~~~~~~~~~~~~~~~~~~~~~~~~~~ Longitudinal forces ~~~~~~~~~~~~~~~~~~~~~~~~~~
Fx_FL = (T_FL.*tau - Tbrk_FL)/rs;
Fx_FR = (T_FR.*tau - Tbrk_FR)/rs;
Fx_RL = (T_RL.*tau - Tbrk_RL)/rs;
Fx_RR = (T_RR.*tau - Tbrk_RR)/rs;

% ~~~~~~~~~~~~~~~~~~~~~~~~~~~ E.o.M. Balance ~~~~~~~~~~~~~~~~~~~~~~~~~~~~~~
X1 = (Fx_FL + Fx_FR).*cos(delta) - (Fy_FL + Fy_FR).*sin(delta);
X2 = Fx_RL + Fx_RR;
deltaX1 = ((Fx_FR - Fx_FL).*cos(delta) - (Fy_FR - Fy_FL).*sin(delta))/2;
deltaX2 = (Fx_RR - Fx_RL)/2;

Y1 = (Fy_FL + Fy_FR).*cos(delta) + (Fx_FL + Fx_FR).*sin(delta);
Y2 = Fy_RL + Fy_RR;

X = X1 + X2 - Faerox;
Y = Y1 + Y2;
N = Y1*a - Y2*b + deltaX1*tf + deltaX2*tr;

% ~~~~~~~~~~~~~~~~~~~~~~~~~~~ System Dynamics f(x,u) ~~~~~~~~~~~~~~~~~~~~~~
xout(1) =  1/m.*(X + vy.*r)*dt + x(1);
xout(2) =  1/m.*(Y - vx.*r)*dt + x(2);
xout(3) =  1/Iz.*(N)*dt + x(3);
end

== matlab function TVModel/Subsystem/Subsystem1/Torque Distribution/MPC/USEFUL STUFFFF/Extended Kalman Filter/measurement_kalman_simulink/h(x) ==
  data: x input; y output
function y = measurement_kalman_simulink(x)

y = zeros(3,1);
y(1) = x(1);
y(2) = x(2);
y(3) = x(3);

end

== stateflow chart TVModel/Subsystem/Subsystem1/Slip Control/Traction Control/TC_Activation_Logic ==
  state TS_ON
    state TC_OFF
      en,du:
      t_max_pid(1:4) = t_limit_positive(1:4);
    state TC_ON
      state FL [parallel]
        settings: executionOrder=1
        state TC_INACTIVE
          en:
          t_max_pid(1) = t_limit_positive(1);
          du:
          t_max_pid(1) = t_limit_positive(1);
        state TC_ACTIVE
          en:
          t_max_pid(1) = abs(t_actual(1));
          du:
          t_max_pid(1) = t_max_pid(1)+t_pid(1);
        (default) -> TS_ON.TC_ON.FL.TC_INACTIVE
        TS_ON.TC_ON.FL.TC_INACTIVE -> TS_ON.TC_ON.FL.TC_ACTIVE : [slip_ratio(1) >= slip_ratio_target]
        TS_ON.TC_ON.FL.TC_ACTIVE -> TS_ON.TC_ON.FL.TC_INACTIVE : [slip_ratio(1) < slip_ratio_target*0.3]
      state FR [parallel]
        settings: executionOrder=2
        state TC_ACTIVE
          en:
          t_max_pid(2) = abs(t_actual(2));
          du:
          t_max_pid(2) = t_max_pid(2)+t_pid(2);
        state TC_INACTIVE
          en:
          t_max_pid(2) = t_limit_positive(2);
          du:
          t_max_pid(2) = t_limit_positive(2);
        (default) -> TS_ON.TC_ON.FR.TC_INACTIVE
        TS_ON.TC_ON.FR.TC_INACTIVE -> TS_ON.TC_ON.FR.TC_ACTIVE : [slip_ratio(2) >= slip_ratio_target]
        TS_ON.TC_ON.FR.TC_ACTIVE -> TS_ON.TC_ON.FR.TC_INACTIVE : [slip_ratio(2) < slip_ratio_target*0.3]
      state RL [parallel]
        settings: executionOrder=3
        state TC_INACTIVE
          en:
          t_max_pid(3) = t_limit_positive(3);
          du:
          t_max_pid(3) = t_limit_positive(3);
        state TC_ACTIVE
          en:
          t_max_pid(3) = abs(t_actual(3));
          du:
          t_max_pid(3) = t_max_pid(3)+t_pid(3);
        (default) -> TS_ON.TC_ON.RL.TC_INACTIVE
        TS_ON.TC_ON.RL.TC_INACTIVE -> TS_ON.TC_ON.RL.TC_ACTIVE : [slip_ratio(3) >= slip_ratio_target]
        TS_ON.TC_ON.RL.TC_ACTIVE -> TS_ON.TC_ON.RL.TC_INACTIVE : [slip_ratio(3) < slip_ratio_target*0.3]
      state RR [parallel]
        settings: executionOrder=4
        state TC_ACTIVE
          en:
          t_max_pid(4) = abs(t_actual(4));
          du:
          t_max_pid(4) = t_max_pid(4)+t_pid(4);
        state TC_INACTIVE
          en:
          t_max_pid(4) = t_limit_positive(4);
          du:
          t_max_pid(4) = t_limit_positive(4);
        (default) -> TS_ON.TC_ON.RR.TC_INACTIVE
        TS_ON.TC_ON.RR.TC_INACTIVE -> TS_ON.TC_ON.RR.TC_ACTIVE : [slip_ratio(4) >= slip_ratio_target]
        TS_ON.TC_ON.RR.TC_ACTIVE -> TS_ON.TC_ON.RR.TC_INACTIVE : [slip_ratio(4) < slip_ratio_target*0.3]
    (default) -> TC_OFF
    TC_ON -> TC_OFF : [tc_flag == 0]
    TC_OFF -> TC_ON : [tc_flag == 1]
  state TS_OFF
    en:
    t_max_pid(1:4) = zeros(4,1);
  (default) -> TS_OFF
  TS_OFF -> TS_ON : [rtd_flag == 1]
  TS_ON -> TS_OFF : [rtd_flag == 0]
  data: t_pid input; t_actual input; rtd_flag input; tc_flag input; t_max_pid output =zeros(4, 1); t_limit_positive input; slip_ratio input; slip_ratio_target input

== matlab function TVModel/Subsystem/Subsystem1/Torque Distribution/Reference Tracking/MATLAB Function1 ==
  data: vx input; u input; y output
function y = fcn(vx,u)

K = 0;
wb = 1.53;

y = u*vx/(wb+K*vx^2);

== matlab function TVModel/Subsystem/Subsystem1/Slip Control/Traction Control/Subsystem/MATLAB Function1 ==
  data: vx input; T_ff output; kappa input; Fz input; kappa_p input; omega_p input; T_ff_deceleration output; T_ff_slip output
function [T_ff,T_ff_deceleration,T_ff_slip] = fcn(vx,kappa,Fz,kappa_p,omega_p)

LMU = 0.93;
J_wheel = 2e5/1e6;
rs = 0.235;
m = 270/4;
tau = 13.5;
dt = 0.02;
g = 9.81;

% @(Fz,LMUX,kappa)
% Old tire
% muX = ((Fz.^2.*LMUX)./1.0e+4-Fz.*LMUX.*sin(atan((Fz.*5.946e-5-6.5736e-1).*(sign(Fz.*(-1.5696e-6)+kappa+6.665e-4).*5.242e-1+1.0).*(atan((Fz.*exp(Fz.*(-1.3455e-5)+1.3455e-2).*(Fz.*(3.0./2.0e+2)+6.77e+2./1.0e+1).*(Fz.*(-1.5696e-6)+kappa+6.665e-4).*(3.33e+2./4.0e+2))./(Fz.*LMUX.*2.5847808+1.0./1.0e+2))-(Fz.*exp(Fz.*(-1.3455e-5)+1.3455e-2).*(Fz.*(3.0./2.0e+2)+6.77e+2./1.0e+1).*(Fz.*(-1.5696e-6)+kappa+6.665e-4).*(3.33e+2./4.0e+2))./(Fz.*LMUX.*2.5847808+1.0./1.0e+2))-(Fz.*exp(Fz.*(-1.3455e-5)+1.3455e-2).*(Fz.*(3.0./2.0e+2)+6.77e+2./1.0e+1).*(Fz.*(-1.5696e-6)+kappa+6.665e-4).*(3.33e+2./4.0e+2))./(Fz.*LMUX.*2.5847808+1.0./1.0e+2)).*(1.68e+2./1.25e+2)).*1.9232)./Fz;

% New tire
muX = (1.0e-4.*Fz.^2.*LMU - 1.92.*Fz.*LMU.*sin(1.41.*atan(0.7.*(5.95e-5.*Fz - 0.657).*(0.524*sign(kappa - 1.57e-6.*Fz + 6.66e-4) + 1.0).*(atan((0.7.*Fz.*exp(0.0135 - 1.35e-5.*Fz).*(0.015.*Fz + 67.7).*(kappa - 1.57e-6.*Fz + 6.66e-4))./(2.71.*Fz.*LMU + 0.01)) - (0.7.*Fz.*exp(0.0135 - 1.35e-5.*Fz).*(0.015.*Fz + 67.7).*(kappa - 1.57e-6.*Fz + 6.66e-4))./(2.71.*Fz.*LMU + 0.01)) - (0.7.*Fz.*exp(0.0135 - 1.35e-5.*Fz).*(0.015.*Fz + 67.7).*(kappa - 1.57e-6.*Fz + 6.66e-4))./(2.71.*Fz.*LMU + 0.01))))./Fz;

T_ff_slip = (kappa_p + 1/vx.*( (1-kappa)/m + rs^2/J_wheel ).*Fz.*muX).*vx.*J_wheel/rs/tau;

eta = - omega_p*rs/g;

T_ff_deceleration = (+rs.^2./J_wheel./g.*muX.*Fz - eta).*J_wheel.*g/rs/tau/2;

% alpha = 0.96;
alpha = 1;

T_ff = T_ff_slip*alpha + T_ff_deceleration*(1 - alpha);

end

== matlab function TVModel/Subsystem/Subsystem1/Torque Distribution/MPC/USEFUL STUFFFF/Non-Linear Activation ==
  data: in_1 input; epsilon input; out output; in_2 input
function out = fcn(in_1,epsilon,in_2)

beta = 4;
epsilon = 1/(1 + (epsilon/(1-epsilon))^(-beta) );

out = in_1*epsilon + in_2*(1 - epsilon) ;

== stateflow chart TVModel/Subsystem/Subsystem1/Torque Distribution/MPC/USEFUL STUFFFF/Chart ==
  state PID_on
    en:
    PID_flag = 1;
  state PID_off
    en:
    PID_flag = 0;
  (default) -> PID_on
  PID_on -> PID_off : [(front_wheels_steering-steer_threshold+semi_amplitude)/(2*semi_amplitude) < 1]
  PID_off -> PID_on : [(front_wheels_steering-steer_threshold+semi_amplitude)/(2*semi_amplitude) > 1]
  data: front_wheels_steering input; semi_amplitude input; PID_flag output; steer_threshold input

== matlab function TVModel/Subsystem/Subsystem1/Torque Distribution/MPC/USEFUL STUFFFF/Yrd 0 When Steering 0/Linear Activation ==
  data: in_1 input; epsilon input; out output; in_2 input
function out = fcn(in_1,epsilon,in_2)

out = in_1*epsilon + in_2*(1 - epsilon) ;

== matlab function TVModel/Subsystem/Subsystem1/Torque Distribution/MPC/Mz Generation/MATLAB Function ==
  data: ubMz output; Mz input; lbMz output
function [ubMz, lbMz] = fcn(Mz)

if sign(Mz) > 0
   lbMz = Mz*0.9;
   ubMz = Mz*1.1;
else
   lbMz = Mz*1.1;
   ubMz = Mz*0.9;
end
